simulink model "sampleModel7214_pp_1_1_mu"  (R2018a)
settings: Solver=VariableStepAuto  StartTime=0.0  StopTime=10.0  RelTol=1e-3
undefined symbols (not defined in the file): DiscIntNeverNeededParam
libraries: simulink x52
(part 2 of 2)

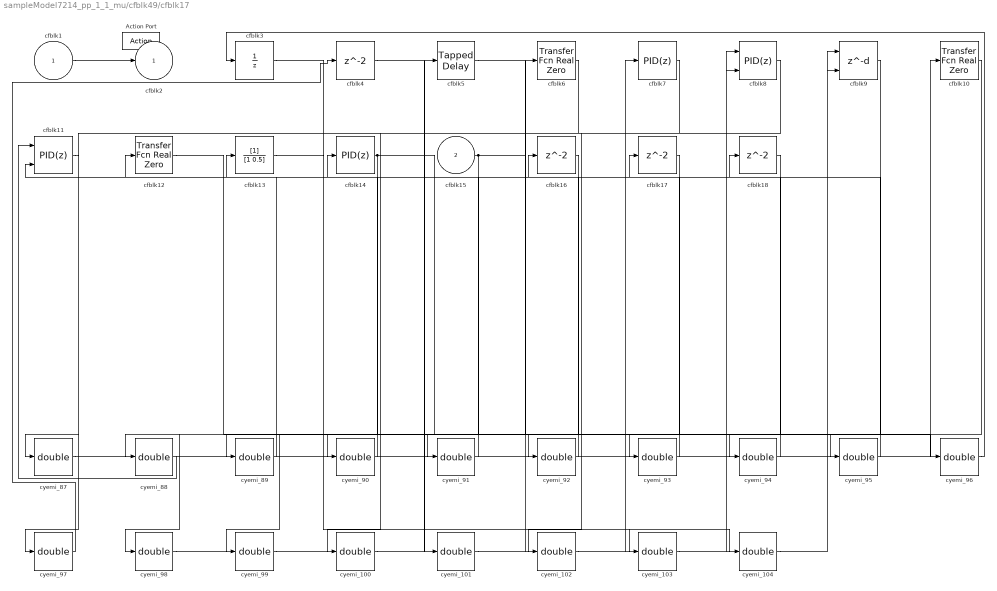
== system sampleModel7214_pp_1_1_mu/cfblk49/cfblk17 ==
  cfblk1 : Inport
  cfblk15 : Inport  Port=2
  Action Port : ActionPort  ActionType=then
  cfblk10 : simulink/Discrete/Transfer Fcn Real Zero  ZeroZ=0.75  ICPrevInput=0.0  DoSatur=off
      settings: SourceProductName=Simulink  SourceProductBaseCode=SL
  cfblk11 : simulink/Continuous/PID Controller (2DOF)  Controller=PID  TimeDomain=Discrete-time  SampleTime=-1  IntegratorMethod=Forward Euler  FilterMethod=Forward Euler  Form=Parallel  UseFilter=on  ControllerParametersSource=internal  P=1  I=1  D=0  N=100  b=1  c=1  InitialConditionSource=internal  InitialConditionForIntegrator=0  InitialConditionForFilter=0  ExternalReset=none  LimitOutput=off  UpperSaturationLimit=inf  LowerSaturationLimit=-inf  LinearizeAsGain=off  AntiWindupMode=none  Kb=1  TrackingMode=off  Kt=1  PParamMin=[]  PParamMax=[]  IParamMin=[]  IParamMax=[]  DParamMin=[]  DParamMax=[]  NParamMin=[]  NParamMax=[]  bParamMin=[]  bParamMax=[]  cParamMin=[]  cParamMax=[]  KbParamMin=[]  KbParamMax=[]  KtParamMin=[]  KtParamMax=[]  POutMin=[]  POutMax=[]  IOutMin=[]  IOutMax=[]  DOutMin=[]  DOutMax=[]  NOutMin=[]  NOutMax=[]  bOutMin=[]  bOutMax=[]  cOutMin=[]  cOutMax=[]  KbOutMin=[]  KbOutMax=[]  KtOutMin=[]  KtOutMax=[]  IntegratorOutMin=[]  IntegratorOutMax=[]  FilterOutMin=[]  FilterOutMax=[]  SumOutMin=[]  SumOutMax=[]  Sum1OutMin=[]  Sum1OutMax=[]  Sum2OutMin=[]  Sum2OutMax=[]  Sum3OutMin=[]  Sum3OutMax=[]  SumI1OutMin=[]  SumI1OutMax=[]  SumI2OutMin=[]  SumI2OutMax=[]  SumI3OutMin=[]  SumI3OutMax=[]  SumDOutMin=[]  SumDOutMax=[]  SaturationOutMin=[]  SaturationOutMax=[]  IntegratorContinuousStateAttributes=''  IntegratorStateMustResolveToSignalObject=off  IntegratorRTWStateStorageClass=Auto  FilterContinuousStateAttributes=''  FilterStateMustResolveToSignalObject=off  FilterRTWStateStorageClass=Auto  DifferentiatorICPrevScaledInput=0  DifferentiatorOutMin=[]  DifferentiatorOutMax=[]  FilterDiffOutCoefMin=[]  FilterDiffOutCoefMax=[]  SumDenOutMin=[]  SumDenOutMax=[]  SumNumOutMin=[]  SumNumOutMax=[]  ReciprocalOutMin=[]  ReciprocalOutMax=[]  DivideOutMin=[]  DivideOutMax=[]  TunerSelectOption=Transfer Function Based (PID Tuner App)
  cfblk12 : simulink/Discrete/Transfer Fcn Real Zero  ZeroZ=0.75  ICPrevInput=0.0  DoSatur=off
      settings: SourceProductName=Simulink  SourceProductBaseCode=SL
  cfblk13 : DiscreteFilter
  cfblk14 : simulink/Continuous/PID Controller  Controller=PID  TimeDomain=Discrete-time  SampleTime=-1  IntegratorMethod=Forward Euler  FilterMethod=Forward Euler  Form=Parallel  UseFilter=on  ControllerParametersSource=internal  P=1  I=1  D=0  N=100  InitialConditionSource=internal  InitialConditionForIntegrator=0  InitialConditionForFilter=0  ExternalReset=none  LimitOutput=off  UpperSaturationLimit=inf  LowerSaturationLimit=-inf  LinearizeAsGain=off  AntiWindupMode=none  Kb=1  TrackingMode=off  Kt=1  PParamMin=[]  PParamMax=[]  IParamMin=[]  IParamMax=[]  DParamMin=[]  DParamMax=[]  NParamMin=[]  NParamMax=[]  KbParamMin=[]  KbParamMax=[]  KtParamMin=[]  KtParamMax=[]  POutMin=[]  POutMax=[]  IOutMin=[]  IOutMax=[]  DOutMin=[]  DOutMax=[]  NOutMin=[]  NOutMax=[]  KbOutMin=[]  KbOutMax=[]  KtOutMin=[]  KtOutMax=[]  IntegratorOutMin=[]  IntegratorOutMax=[]  FilterOutMin=[]  FilterOutMax=[]  SumOutMin=[]  SumOutMax=[]  SumI1OutMin=[]  SumI1OutMax=[]  SumI2OutMin=[]  SumI2OutMax=[]  SumI3OutMin=[]  SumI3OutMax=[]  SumDOutMin=[]  SumDOutMax=[]  SaturationOutMin=[]  SaturationOutMax=[]  IntegratorContinuousStateAttributes=''  IntegratorStateMustResolveToSignalObject=off  IntegratorRTWStateStorageClass=Auto  FilterContinuousStateAttributes=''  FilterStateMustResolveToSignalObject=off  FilterRTWStateStorageClass=Auto  DifferentiatorICPrevScaledInput=0  DifferentiatorOutMin=[]  DifferentiatorOutMax=[]  FilterDiffOutCoefMin=[]  FilterDiffOutCoefMax=[]  SumDenOutMin=[]  SumDenOutMax=[]  SumNumOutMin=[]  SumNumOutMax=[]  ReciprocalOutMin=[]  ReciprocalOutMax=[]  DivideOutMin=[]  DivideOutMax=[]  TunerSelectOption=Transfer Function Based (PID Tuner App)
  cfblk{4,16..18} (4 alike) : Delay
  cfblk3 : UnitDelay  SampleTime=-1
  cfblk5 : simulink/Discrete/Tapped Delay  vinit=0.0  samptime=-1  NumDelays=1  DelayOrder=Oldest  includeCurrent=off
  cfblk6 : simulink/Discrete/Transfer Fcn Real Zero  ZeroZ=0.75  ICPrevInput=0.0  DoSatur=off
      settings: SourceProductName=Simulink  SourceProductBaseCode=SL
  cfblk7 : simulink/Continuous/PID Controller  Controller=PID  TimeDomain=Discrete-time  SampleTime=-1  IntegratorMethod=Forward Euler  FilterMethod=Forward Euler  Form=Parallel  UseFilter=on  ControllerParametersSource=internal  P=1  I=1  D=0  N=100  InitialConditionSource=internal  InitialConditionForIntegrator=0  InitialConditionForFilter=0  ExternalReset=none  LimitOutput=off  UpperSaturationLimit=inf  LowerSaturationLimit=-inf  LinearizeAsGain=off  AntiWindupMode=none  Kb=1  TrackingMode=off  Kt=1  PParamMin=[]  PParamMax=[]  IParamMin=[]  IParamMax=[]  DParamMin=[]  DParamMax=[]  NParamMin=[]  NParamMax=[]  KbParamMin=[]  KbParamMax=[]  KtParamMin=[]  KtParamMax=[]  POutMin=[]  POutMax=[]  IOutMin=[]  IOutMax=[]  DOutMin=[]  DOutMax=[]  NOutMin=[]  NOutMax=[]  KbOutMin=[]  KbOutMax=[]  KtOutMin=[]  KtOutMax=[]  IntegratorOutMin=[]  IntegratorOutMax=[]  FilterOutMin=[]  FilterOutMax=[]  SumOutMin=[]  SumOutMax=[]  SumI1OutMin=[]  SumI1OutMax=[]  SumI2OutMin=[]  SumI2OutMax=[]  SumI3OutMin=[]  SumI3OutMax=[]  SumDOutMin=[]  SumDOutMax=[]  SaturationOutMin=[]  SaturationOutMax=[]  IntegratorContinuousStateAttributes=''  IntegratorStateMustResolveToSignalObject=off  IntegratorRTWStateStorageClass=Auto  FilterContinuousStateAttributes=''  FilterStateMustResolveToSignalObject=off  FilterRTWStateStorageClass=Auto  DifferentiatorICPrevScaledInput=0  DifferentiatorOutMin=[]  DifferentiatorOutMax=[]  FilterDiffOutCoefMin=[]  FilterDiffOutCoefMax=[]  SumDenOutMin=[]  SumDenOutMax=[]  SumNumOutMin=[]  SumNumOutMax=[]  ReciprocalOutMin=[]  ReciprocalOutMax=[]  DivideOutMin=[]  DivideOutMax=[]  TunerSelectOption=Transfer Function Based (PID Tuner App)
  cfblk8 : simulink/Continuous/PID Controller (2DOF)  Controller=PID  TimeDomain=Discrete-time  SampleTime=-1  IntegratorMethod=Forward Euler  FilterMethod=Forward Euler  Form=Parallel  UseFilter=on  ControllerParametersSource=internal  P=1  I=1  D=0  N=100  b=1  c=1  InitialConditionSource=internal  InitialConditionForIntegrator=0  InitialConditionForFilter=0  ExternalReset=none  LimitOutput=off  UpperSaturationLimit=inf  LowerSaturationLimit=-inf  LinearizeAsGain=off  AntiWindupMode=none  Kb=1  TrackingMode=off  Kt=1  PParamMin=[]  PParamMax=[]  IParamMin=[]  IParamMax=[]  DParamMin=[]  DParamMax=[]  NParamMin=[]  NParamMax=[]  bParamMin=[]  bParamMax=[]  cParamMin=[]  cParamMax=[]  KbParamMin=[]  KbParamMax=[]  KtParamMin=[]  KtParamMax=[]  POutMin=[]  POutMax=[]  IOutMin=[]  IOutMax=[]  DOutMin=[]  DOutMax=[]  NOutMin=[]  NOutMax=[]  bOutMin=[]  bOutMax=[]  cOutMin=[]  cOutMax=[]  KbOutMin=[]  KbOutMax=[]  KtOutMin=[]  KtOutMax=[]  IntegratorOutMin=[]  IntegratorOutMax=[]  FilterOutMin=[]  FilterOutMax=[]  SumOutMin=[]  SumOutMax=[]  Sum1OutMin=[]  Sum1OutMax=[]  Sum2OutMin=[]  Sum2OutMax=[]  Sum3OutMin=[]  Sum3OutMax=[]  SumI1OutMin=[]  SumI1OutMax=[]  SumI2OutMin=[]  SumI2OutMax=[]  SumI3OutMin=[]  SumI3OutMax=[]  SumDOutMin=[]  SumDOutMax=[]  SaturationOutMin=[]  SaturationOutMax=[]  IntegratorContinuousStateAttributes=''  IntegratorStateMustResolveToSignalObject=off  IntegratorRTWStateStorageClass=Auto  FilterContinuousStateAttributes=''  FilterStateMustResolveToSignalObject=off  FilterRTWStateStorageClass=Auto  DifferentiatorICPrevScaledInput=0  DifferentiatorOutMin=[]  DifferentiatorOutMax=[]  FilterDiffOutCoefMin=[]  FilterDiffOutCoefMax=[]  SumDenOutMin=[]  SumDenOutMax=[]  SumNumOutMin=[]  SumNumOutMax=[]  ReciprocalOutMin=[]  ReciprocalOutMax=[]  DivideOutMin=[]  DivideOutMax=[]  TunerSelectOption=Transfer Function Based (PID Tuner App)
  cfblk9 : Delay  DelayLengthSource=Input port
      settings: InputPortMap=u0,p1
  cyemi_{87..104} (18 alike) : DataTypeConversion  OutDataTypeStr=double
  cfblk2 : Outport
  wires:
  cfblk14/1 -> cyemi_93/1, cyemi_98/1
  cfblk1/1 -> cfblk2/1
  cfblk15/1 -> cyemi_91/1, cyemi_96/1
  cyemi_87/1 -> cfblk10/1
  cfblk8/1 -> cyemi_87/1
  cyemi_88/1 -> cfblk11/1
  cfblk16/1 -> cyemi_88/1
  cyemi_89/1 -> cfblk11/2
  cfblk9/1 -> cyemi_89/1
  cyemi_90/1 -> cfblk12/1
  cfblk6/1 -> cyemi_90/1
  cyemi_91/1 -> cfblk13/1
  cyemi_92/1 -> cfblk14/1
  cfblk7/1 -> cyemi_92/1
  cyemi_93/1 -> cfblk16/1
  cyemi_94/1 -> cfblk17/1
  cfblk5/1 -> cyemi_94/1
  cyemi_95/1 -> cfblk18/1
  cfblk12/1 -> cyemi_95/1
  cyemi_96/1 -> cfblk3/1
  cyemi_97/1 -> cfblk4/1
  cfblk11/1 -> cyemi_97/1
  cyemi_98/1 -> cfblk5/1
  cyemi_99/1 -> cfblk6/1
  cfblk18/1 -> cyemi_99/1
  cyemi_100/1 -> cfblk7/1
  cfblk10/1 -> cyemi_100/1
  cyemi_101/1 -> cfblk8/1
  cfblk4/1 -> cyemi_101/1
  cyemi_102/1 -> cfblk8/2
  cfblk17/1 -> cyemi_102/1
  cyemi_103/1 -> cfblk9/1
  cfblk3/1 -> cyemi_103/1
  cyemi_104/1 -> cfblk9/2
  cfblk13/1 -> cyemi_104/1

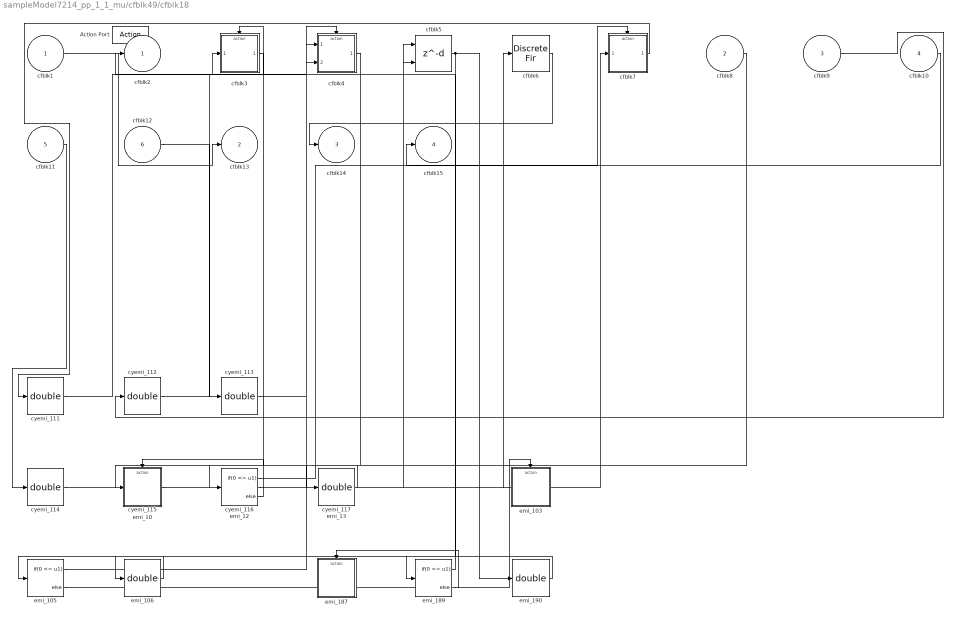
== system sampleModel7214_pp_1_1_mu/cfblk49/cfblk18 ==
  cfblk1 : Inport
  cfblk8 : Inport  Port=2
  cfblk9 : Inport  Port=3
  cfblk10 : Inport  Port=4
  cfblk11 : Inport  Port=5
  cfblk12 : Inport  Port=6
  Action Port : ActionPort  ActionType=else
  cfblk3 : Subsystem  TreatAsAtomicUnit=on
  cfblk4 : Subsystem  TreatAsAtomicUnit=on
  cfblk5 : Delay  DelayLengthSource=Input port
      settings: InputPortMap=u0,p1
  cfblk6 : DiscreteFir
  cfblk7 : Subsystem  TreatAsAtomicUnit=on
  cyemi_{111..117} (7 alike) : DataTypeConversion  OutDataTypeStr=double
  emi_10 : Subsystem  TreatAsAtomicUnit=on
  emi_103 : Subsystem  TreatAsAtomicUnit=on
  emi_105 : If  IfExpression=0 <= u1
  emi_106 : DataTypeConversion  OutDataTypeStr=double
  emi_12 : If  IfExpression=0 <= u1
  emi_13 : DataTypeConversion  OutDataTypeStr=double
  emi_187 : Subsystem  TreatAsAtomicUnit=on
  emi_189 : If  IfExpression=0 <= u1
  emi_190 : DataTypeConversion  OutDataTypeStr=double
  cfblk2 : Outport
  cfblk13 : Outport  Port=2
  cfblk14 : Outport  Port=3
  cfblk15 : Outport  Port=4
  wires:
  cfblk1/1 -> cfblk13/1
  cfblk6/1 -> cfblk14/1
  cfblk5/1 -> cfblk2/1, emi_13/1, emi_106/1, emi_190/1
  cfblk10/1 -> cfblk15/1
  cfblk9/1 -> cyemi_112/1
  cfblk12/1 -> cyemi_113/1
  cyemi_114/1 -> cfblk5/1
  cfblk11/1 -> cyemi_114/1
  cyemi_115/1 -> cfblk5/2
  cfblk8/1 -> cyemi_115/1
  cyemi_116/1 -> cfblk6/1
  cyemi_117/1 -> cfblk7/1(emi_8)
  cfblk7/1(emi_9) -> cyemi_111/1
  emi_12/1 -> cfblk7/Action
  emi_12/2 -> emi_10/Action
  emi_13/1 -> emi_12/1
  cyemi_112/1 -> cfblk4/1(emi_100)
  cyemi_113/1 -> cfblk4/2(emi_101)
  cfblk4/1(emi_102) -> cyemi_117/1
  emi_105/1 -> cfblk4/Action
  emi_105/2 -> emi_103/Action
  emi_106/1 -> emi_105/1
  cyemi_111/1 -> cfblk3/1(emi_185)
  cfblk3/1(emi_186) -> cyemi_116/1
  emi_189/1 -> cfblk3/Action
  emi_189/2 -> emi_187/Action
  emi_190/1 -> emi_189/1

== system sampleModel7214_pp_1_1_mu/cfblk49/cfblk21 ==
  emi_64 : Inport
  Action Port : ActionPort  ActionType=then
  cfblk21 : Delay
  emi_65 : Outport
  wires:
  emi_64/1 -> cfblk21/1
  cfblk21/1 -> emi_65/1

== system sampleModel7214_pp_1_1_mu/cfblk49/cfblk24 ==
  emi_157 : Inport
  Action Port : ActionPort  ActionType=then
  cfblk24 : Delay
  emi_158 : Outport
  wires:
  emi_157/1 -> cfblk24/1
  cfblk24/1 -> emi_158/1

== system sampleModel7214_pp_1_1_mu/cfblk49/cfblk4 ==
  emi_150 : Inport
  Action Port : ActionPort  ActionType=then
  cfblk4 : UnitDelay  SampleTime=-1
  emi_151 : Outport
  wires:
  emi_150/1 -> cfblk4/1
  cfblk4/1 -> emi_151/1

== system sampleModel7214_pp_1_1_mu/cfblk49/cfblk5 ==
  emi_178 : Inport
  Action Port : ActionPort  ActionType=then
  cfblk5 : simulink/Continuous/PID Controller  Controller=PID  TimeDomain=Discrete-time  SampleTime=-1  IntegratorMethod=Forward Euler  FilterMethod=Forward Euler  Form=Parallel  UseFilter=on  ControllerParametersSource=internal  P=1  I=1  D=0  N=100  InitialConditionSource=internal  InitialConditionForIntegrator=0  InitialConditionForFilter=0  ExternalReset=none  LimitOutput=off  UpperSaturationLimit=inf  LowerSaturationLimit=-inf  LinearizeAsGain=off  AntiWindupMode=none  Kb=1  TrackingMode=off  Kt=1  PParamMin=[]  PParamMax=[]  IParamMin=[]  IParamMax=[]  DParamMin=[]  DParamMax=[]  NParamMin=[]  NParamMax=[]  KbParamMin=[]  KbParamMax=[]  KtParamMin=[]  KtParamMax=[]  POutMin=[]  POutMax=[]  IOutMin=[]  IOutMax=[]  DOutMin=[]  DOutMax=[]  NOutMin=[]  NOutMax=[]  KbOutMin=[]  KbOutMax=[]  KtOutMin=[]  KtOutMax=[]  IntegratorOutMin=[]  IntegratorOutMax=[]  FilterOutMin=[]  FilterOutMax=[]  SumOutMin=[]  SumOutMax=[]  SumI1OutMin=[]  SumI1OutMax=[]  SumI2OutMin=[]  SumI2OutMax=[]  SumI3OutMin=[]  SumI3OutMax=[]  SumDOutMin=[]  SumDOutMax=[]  SaturationOutMin=[]  SaturationOutMax=[]  IntegratorContinuousStateAttributes=''  IntegratorStateMustResolveToSignalObject=off  IntegratorRTWStateStorageClass=Auto  FilterContinuousStateAttributes=''  FilterStateMustResolveToSignalObject=off  FilterRTWStateStorageClass=Auto  DifferentiatorICPrevScaledInput=0  DifferentiatorOutMin=[]  DifferentiatorOutMax=[]  FilterDiffOutCoefMin=[]  FilterDiffOutCoefMax=[]  SumDenOutMin=[]  SumDenOutMax=[]  SumNumOutMin=[]  SumNumOutMax=[]  ReciprocalOutMin=[]  ReciprocalOutMax=[]  DivideOutMin=[]  DivideOutMax=[]  TunerSelectOption=Transfer Function Based (PID Tuner App)
  emi_179 : Outport
  wires:
  emi_178/1 -> cfblk5/1
  cfblk5/1 -> emi_179/1

== system sampleModel7214_pp_1_1_mu/cfblk49/cfblk8 ==
  emi_50 : Inport
  Action Port : ActionPort  ActionType=then
  cfblk8 : Delay
  emi_51 : Outport
  wires:
  emi_50/1 -> cfblk8/1
  cfblk8/1 -> emi_51/1

== system sampleModel7214_pp_1_1_mu/cfblk49/emi_152 ==
  Action Port : ActionPort  ActionType=else
  emi_153 : Assertion

== system sampleModel7214_pp_1_1_mu/cfblk49/emi_159 ==
  Action Port : ActionPort  ActionType=else
  emi_160 : Assertion

== system sampleModel7214_pp_1_1_mu/cfblk49/emi_180 ==
  Action Port : ActionPort  ActionType=else
  emi_181 : Assertion

== system sampleModel7214_pp_1_1_mu/cfblk49/emi_52 ==
  Action Port : ActionPort  ActionType=else
  emi_53 : Assertion

== system sampleModel7214_pp_1_1_mu/cfblk49/emi_66 ==
  Action Port : ActionPort  ActionType=else
  emi_67 : Assertion

== system sampleModel7214_pp_1_1_mu/cfblk49/emi_73 ==
  Action Port : ActionPort  ActionType=else
  emi_74 : Assertion

== system sampleModel7214_pp_1_1_mu/cfblk50/cfblk5 ==
  emi_1 : Inport
  Action Port : ActionPort  ActionType=then
  cfblk5 : simulink/Discrete/Difference  ICPrevInput=0.0  OutMin=[]  OutMax=[]  OutDataTypeStr=double  OutputDataTypeScalingMode=double  OutDataType=fixdt(1, 16)  OutScaling=2^-10  DoSatur=off
  emi_2 : Outport
  wires:
  emi_1/1 -> cfblk5/1
  cfblk5/1 -> emi_2/1

== system sampleModel7214_pp_1_1_mu/cfblk50/cfblk7 ==
  emi_78 : Inport
  Action Port : ActionPort  ActionType=then
  cfblk7 : DiscreteIntegrator  SampleTime=-1  OutDataTypeStr=double  ICPrevOutput=DiscIntNeverNeededParam  ICPrevScaledInput=DiscIntNeverNeededParam
  emi_79 : Outport
  wires:
  emi_78/1 -> cfblk7/1
  cfblk7/1 -> emi_79/1

== system sampleModel7214_pp_1_1_mu/cfblk50/emi_3 ==
  Action Port : ActionPort  ActionType=else
  emi_4 : Assertion

== system sampleModel7214_pp_1_1_mu/cfblk50/emi_80 ==
  Action Port : ActionPort  ActionType=else
  emi_81 : Assertion

== system sampleModel7214_pp_1_1_mu/cfblk52/cfblk5 ==
  emi_207 : Inport
  Action Port : ActionPort  ActionType=then
  cfblk5 : DiscreteTransferFcn
  emi_208 : Outport
  wires:
  emi_207/1 -> cfblk5/1
  cfblk5/1 -> emi_208/1

== system sampleModel7214_pp_1_1_mu/cfblk52/cfblk9 ==
  emi_22 : Inport
  Action Port : ActionPort  ActionType=then
  cfblk9 : DiscreteZeroPole  Poles=[0 0.5]  Gain=1  SampleTime=-1
  emi_23 : Outport
  wires:
  emi_22/1 -> cfblk9/1
  cfblk9/1 -> emi_23/1

== system sampleModel7214_pp_1_1_mu/cfblk52/emi_209 ==
  Action Port : ActionPort  ActionType=else
  emi_210 : Assertion

== system sampleModel7214_pp_1_1_mu/cfblk52/emi_24 ==
  Action Port : ActionPort  ActionType=else
  emi_25 : Assertion

== system sampleModel7214_pp_1_1_mu/cfblk53/cfblk12 ==
  emi_57 : Inport
  Action Port : ActionPort  ActionType=then
  cfblk12 : Delay
  emi_58 : Outport
  wires:
  emi_57/1 -> cfblk12/1
  cfblk12/1 -> emi_58/1

== system sampleModel7214_pp_1_1_mu/cfblk53/cfblk7 ==
  emi_15 : Inport
  Action Port : ActionPort  ActionType=then
  cfblk7 : Delay
  emi_16 : Outport
  wires:
  emi_15/1 -> cfblk7/1
  cfblk7/1 -> emi_16/1

== system sampleModel7214_pp_1_1_mu/cfblk53/emi_17 ==
  Action Port : ActionPort  ActionType=else
  emi_18 : Assertion

== system sampleModel7214_pp_1_1_mu/cfblk53/emi_59 ==
  Action Port : ActionPort  ActionType=else
  emi_60 : Assertion

== system sampleModel7214_pp_1_1_mu/cfblk48/cfblk16/cfblk10 ==
  emi_36 : Inport
  Action Port : ActionPort  ActionType=then
  cfblk10 : DiscreteZeroPole  Poles=[0 0.5]  Gain=1  SampleTime=-1
  emi_37 : Outport
  wires:
  emi_36/1 -> cfblk10/1
  cfblk10/1 -> emi_37/1

== system sampleModel7214_pp_1_1_mu/cfblk48/cfblk16/cfblk18 ==
  emi_29 : Inport
  Action Port : ActionPort  ActionType=then
  cfblk18 : Delay
  emi_30 : Outport
  wires:
  emi_29/1 -> cfblk18/1
  cfblk18/1 -> emi_30/1

== system sampleModel7214_pp_1_1_mu/cfblk48/cfblk16/emi_31 ==
  Action Port : ActionPort  ActionType=else
  emi_32 : Assertion

== system sampleModel7214_pp_1_1_mu/cfblk48/cfblk16/emi_38 ==
  Action Port : ActionPort  ActionType=else
  emi_39 : Assertion

== system sampleModel7214_pp_1_1_mu/cfblk48/cfblk17/cfblk7 ==
  emi_122 : Inport
  Action Port : ActionPort  ActionType=then
  cfblk7 : DiscreteZeroPole  Poles=[0 0.5]  Gain=1  SampleTime=-1
  emi_123 : Outport
  wires:
  emi_122/1 -> cfblk7/1
  cfblk7/1 -> emi_123/1

== system sampleModel7214_pp_1_1_mu/cfblk48/cfblk17/cfblk8 ==
  emi_164 : Inport
  Action Port : ActionPort  ActionType=then
  cfblk8 : DiscreteFir
  emi_165 : Outport
  wires:
  emi_164/1 -> cfblk8/1
  cfblk8/1 -> emi_165/1

== system sampleModel7214_pp_1_1_mu/cfblk48/cfblk17/emi_124 ==
  Action Port : ActionPort  ActionType=else
  emi_125 : Assertion

== system sampleModel7214_pp_1_1_mu/cfblk48/cfblk17/emi_166 ==
  Action Port : ActionPort  ActionType=else
  emi_167 : Assertion

== system sampleModel7214_pp_1_1_mu/cfblk49/cfblk18/cfblk3 ==
  emi_185 : Inport
  Action Port : ActionPort  ActionType=then
  cfblk3 : simulink/Discrete/Transfer Fcn Lead or Lag  PoleZ=0.95  ZeroZ=0.75  ICPrevOutput=0.0  ICPrevInput=0.0  DoSatur=off
      settings: SourceProductName=Simulink  SourceProductBaseCode=SL
  emi_186 : Outport
  wires:
  emi_185/1 -> cfblk3/1
  cfblk3/1 -> emi_186/1

== system sampleModel7214_pp_1_1_mu/cfblk49/cfblk18/cfblk4 ==
  emi_100 : Inport
  emi_101 : Inport  Port=2
  Action Port : ActionPort  ActionType=then
  cfblk4 : simulink/Continuous/PID Controller (2DOF)  Controller=PID  TimeDomain=Discrete-time  SampleTime=-1  IntegratorMethod=Forward Euler  FilterMethod=Forward Euler  Form=Parallel  UseFilter=on  ControllerParametersSource=internal  P=1  I=1  D=0  N=100  b=1  c=1  InitialConditionSource=internal  InitialConditionForIntegrator=0  InitialConditionForFilter=0  ExternalReset=none  LimitOutput=off  UpperSaturationLimit=inf  LowerSaturationLimit=-inf  LinearizeAsGain=off  AntiWindupMode=none  Kb=1  TrackingMode=off  Kt=1  PParamMin=[]  PParamMax=[]  IParamMin=[]  IParamMax=[]  DParamMin=[]  DParamMax=[]  NParamMin=[]  NParamMax=[]  bParamMin=[]  bParamMax=[]  cParamMin=[]  cParamMax=[]  KbParamMin=[]  KbParamMax=[]  KtParamMin=[]  KtParamMax=[]  POutMin=[]  POutMax=[]  IOutMin=[]  IOutMax=[]  DOutMin=[]  DOutMax=[]  NOutMin=[]  NOutMax=[]  bOutMin=[]  bOutMax=[]  cOutMin=[]  cOutMax=[]  KbOutMin=[]  KbOutMax=[]  KtOutMin=[]  KtOutMax=[]  IntegratorOutMin=[]  IntegratorOutMax=[]  FilterOutMin=[]  FilterOutMax=[]  SumOutMin=[]  SumOutMax=[]  Sum1OutMin=[]  Sum1OutMax=[]  Sum2OutMin=[]  Sum2OutMax=[]  Sum3OutMin=[]  Sum3OutMax=[]  SumI1OutMin=[]  SumI1OutMax=[]  SumI2OutMin=[]  SumI2OutMax=[]  SumI3OutMin=[]  SumI3OutMax=[]  SumDOutMin=[]  SumDOutMax=[]  SaturationOutMin=[]  SaturationOutMax=[]  IntegratorContinuousStateAttributes=''  IntegratorStateMustResolveToSignalObject=off  IntegratorRTWStateStorageClass=Auto  FilterContinuousStateAttributes=''  FilterStateMustResolveToSignalObject=off  FilterRTWStateStorageClass=Auto  DifferentiatorICPrevScaledInput=0  DifferentiatorOutMin=[]  DifferentiatorOutMax=[]  FilterDiffOutCoefMin=[]  FilterDiffOutCoefMax=[]  SumDenOutMin=[]  SumDenOutMax=[]  SumNumOutMin=[]  SumNumOutMax=[]  ReciprocalOutMin=[]  ReciprocalOutMax=[]  DivideOutMin=[]  DivideOutMax=[]  TunerSelectOption=Transfer Function Based (PID Tuner App)
  emi_102 : Outport
  wires:
  emi_100/1 -> cfblk4/1
  emi_101/1 -> cfblk4/2
  cfblk4/1 -> emi_102/1

== system sampleModel7214_pp_1_1_mu/cfblk49/cfblk18/cfblk7 ==
  emi_8 : Inport
  Action Port : ActionPort  ActionType=then
  cfblk7 : simulink/Discrete/Difference  ICPrevInput=0.0  OutMin=[]  OutMax=[]  OutDataTypeStr=double  OutputDataTypeScalingMode=double  OutDataType=fixdt(1, 16)  OutScaling=2^-10  DoSatur=off
  emi_9 : Outport
  wires:
  emi_8/1 -> cfblk7/1
  cfblk7/1 -> emi_9/1

== system sampleModel7214_pp_1_1_mu/cfblk49/cfblk18/emi_10 ==
  Action Port : ActionPort  ActionType=else
  emi_11 : Assertion

== system sampleModel7214_pp_1_1_mu/cfblk49/cfblk18/emi_103 ==
  Action Port : ActionPort  ActionType=else
  emi_104 : Assertion

== system sampleModel7214_pp_1_1_mu/cfblk49/cfblk18/emi_187 ==
  Action Port : ActionPort  ActionType=else
  emi_188 : Assertion
